simulink model "magField_test"  (R2018b)
settings: Solver=VariableStepAuto  StartTime=0.0  StopTime=10.0  RelTol=1e-3
undefined symbols (not defined in the file or in its folder): simParams
libraries: clock_lib x1, time_Lib x1, magField_lib x1
settings Model: Creator=Taylor  LastModifiedBy=taylorreynolds

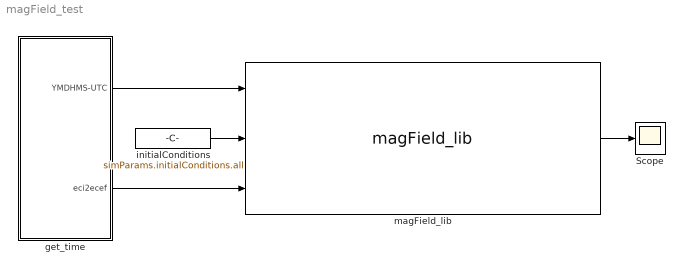
== system magField_test ==
  Scope : Scope
  get_time : Subsystem
  initialConditions : Constant  Value=simParams.initialConditions.all
  magField_lib : magField_lib/magField_lib  SystemSampleTime=-1
  wires:
  get_time/2(eci2ecef) -> magField_lib/3
  get_time/1(YMDHMS-UTC) -> magField_lib/1
  initialConditions/1 -> magField_lib/2
  magField_lib/1 -> Scope/1

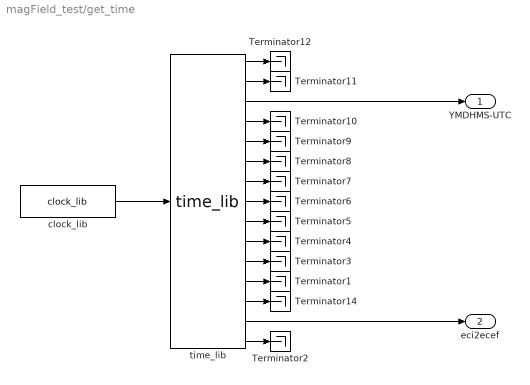
== system magField_test/get_time ==
  Terminator{1..12,14} (13 alike) : Terminator
  clock_lib : clock_lib/clock_lib  SystemSampleTime=-1
  "time_lib " : time_Lib/time_lib    SystemSampleTime=-1
  YMDHMS-UTC : Outport
  eci2ecef : Outport  Port=2
  wires:
  clock_lib/1 -> "time_lib "/1
  "time_lib "/3 -> YMDHMS-UTC/1
  "time_lib "/14 -> eci2ecef/1
  "time_lib "/13 -> Terminator14/1
  "time_lib "/12 -> Terminator1/1
  "time_lib "/15 -> Terminator2/1
  "time_lib "/11 -> Terminator3/1
  "time_lib "/10 -> Terminator4/1
  "time_lib "/9 -> Terminator5/1
  "time_lib "/8 -> Terminator6/1
  "time_lib "/7 -> Terminator7/1
  "time_lib "/6 -> Terminator8/1
  "time_lib "/5 -> Terminator9/1
  "time_lib "/4 -> Terminator10/1
  "time_lib "/2 -> Terminator11/1
  "time_lib "/1 -> Terminator12/1
